simulink model "RefModel_2024"  (R2025b)
settings: Solver=VariableStepAuto  StartTime=0.0  StopTime=10.0  RelTol=1e-3
libraries: aerolibasang x3, simulink_extras x2, aerolibatmos2 x1
settings Model: Creator=Ranvir  LastModifiedBy=ranvirsingh

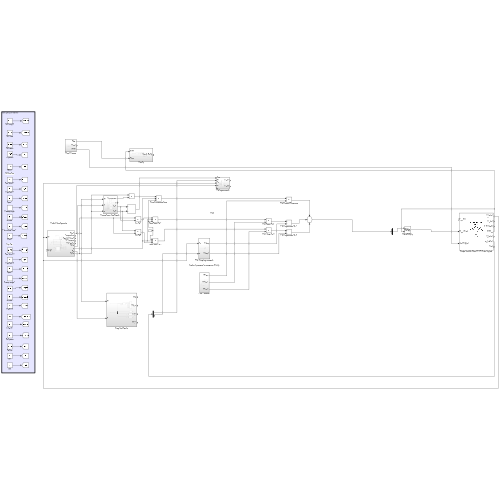
[thumbnail: Simulink's stored preview of the top-level diagram]
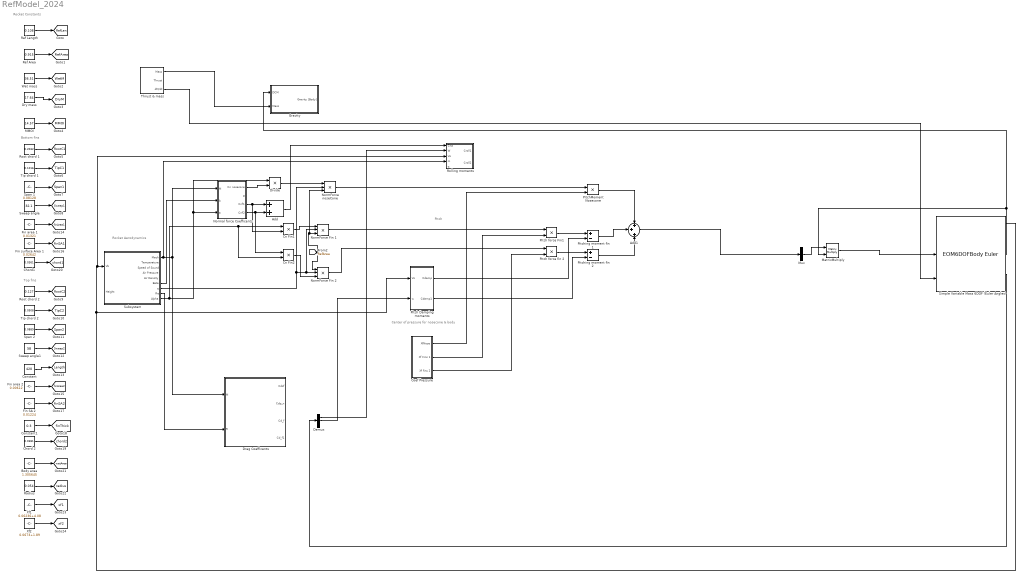
== system RefModel_2024 ==
  note: Center of pressure for nosecone & body
  note: Pitch
  note: Rocket Aerodynamics
  note: Bottom fins
  note: Rocket Constants
  note: Top fins
  Add : Sum
  Add1 : Sum  Inputs=+++
  Body area : Constant  Value=1.305645
  Chord 2 : Constant  Value=0.0381
  Chord1 : Constant  Value=0.0361
  Cn Fin1 : Product  Inputs=**
  Cn Fin2 : Product  Inputs=**
  Coef Pressure : Subsystem
  Constant : Constant  Value=420
  Constant1 : Constant  Value=0.3
  Demux : Demux  Outputs=3
  Divide : Product  Inputs=**
  Drag Coefficents : Subsystem
  Dry mass : Constant  Value=17.64
  Fin SA 2 : Constant  Value=0.01224
  Fin area 1 : Constant  Value=0.01321
  Fin area 2 : Constant  Value=0.00612
  Fin surface Area 1 : Constant  Value=0.02642
  Gravity : Subsystem
  MMOI : Constant  Value=14.57
  MatrixMultiply : Product  Multiplication=Matrix(*)
  Mux : Mux  Inputs=3
  NormForce Fin 1 : Product  Inputs=***
  NormForce Fin 2 : Product  Inputs=***
  NormForce noseCone : Product  Inputs=***
  Normal force Coefficents : Subsystem
  Pitch Damping moments : Subsystem
  Pitch force Fin1 : Product  Inputs=**
  Pitch force fin 2 : Product  Inputs=**
  PitchMoment Nosecone : Product  Inputs=**
  Pitching moment fin 1 : Sum  Inputs=+-
  Pitching moment fin 2 : Sum  Inputs=+-
  Radius : Constant  Value=0.054
  Ref Area : Constant  Value=0.915
  Ref Length : Constant  Value=0.108
  Rolling moments : Subsystem
  Root chord 1 : Constant  Value=0.2032
  Root chord 2 : Constant  Value=0.127
  Simple Variable Mass 6DOF (Euler Angles) : EOM6DOFBodyEuler  mtype=Simple Variable
  Span 1 : Constant  Value=0.08128
  Span 2 : Constant  Value=0.0889
  Subsystem : Subsystem
  Sweep angle : Constant  Value=32.1
  Sweep angle1 : Constant  Value=58
  Thrust & mass : Subsystem
  Tip chord 1 : Constant  Value=0.1016
  Tip chord 2 : Constant  Value=0.0508
  Wet mass : Constant  Value=36.51
  Xf1 : Constant  Value=0.06236+4.08
  Xf2 : Constant  Value=0.0673+1.89
  tag scope: DryM=global, Length=global, MMOI=global, RefArea=global, RefLen=global, RootC1=global, RootC2=global, Span1=global, Span2=global, Sweep1=global, Sweep2=global, TipC1=global, TipC2=global, WetM=global, chord1=global, chord2=global, finArea1=global, finArea2=global, finSA1=global, finSA2=global, finThick=global, radius=global, wetArea=global, xf1=global, xf2=global
  wires:
  Ref Length/1 -> [RefLen]
  Ref Area/1 -> [RefArea]
  Wet mass/1 -> [WetM]
  Dry mass/1 -> [DryM]
  MMOI/1 -> [MMOI]
  Root chord 1/1 -> [RootC1]
  Tip chord 1/1 -> [TipC1]
  Span 1/1 -> [Span1]
  Sweep angle/1 -> [Sweep1]
  Root chord 2/1 -> [RootC2]
  Tip chord 2/1 -> [TipC2]
  Span 2/1 -> [Span2]
  Sweep angle1/1 -> [Sweep2]
  Thrust & mass/1(Mass) -> Gravity/2(Mass)
  Simple Variable Mass 6DOF (Euler Angles)/4 -> MatrixMultiply/2, Gravity/1(DCM)
  Thrust & mass/3(dM/dt) -> Simple Variable Mass 6DOF (Euler Angles)/3
  Constant/1 -> [Length]
  Simple Variable Mass 6DOF (Euler Angles)/1 -> Pitch Damping moments/1(Vo), Rolling moments/3(Vo), Subsystem/1(Vb)
  Fin area 1/1 -> [finArea1]
  Fin area 2/1 -> [finArea2]
  Fin surface Area 1/1 -> [finSA1]
  Fin SA 2/1 -> [finSA2]
  Subsystem/1(Mach) -> Rolling moments/4(m), Drag Coefficents/1(M), Normal force Coefficents/1(M)
  Constant1/1 -> [finThick]
  Chord 2/1 -> [chord2]
  Chord1/1 -> [chord1]
  Body area/1 -> [wetArea]
  Subsystem/8(Re) -> Drag Coefficents/2(R)
  Subsystem/6(Beta) -> Normal force Coefficents/2(b)
  Subsystem/9(Alpha) -> Cn Fin2/2, Cn Fin1/1, Divide/1, Normal force Coefficents/3(a)
  Normal force Coefficents/3(Cnf1) -> Cn Fin1/2, Add/1
  Normal force Coefficents/4(Cnf2) -> Cn Fin2/1, Add/2
  Radius/1 -> [radius]
  Add/1 -> Rolling moments/1(Cna)
  Simple Variable Mass 6DOF (Euler Angles)/6 -> Demux/1
  Xf1/1 -> [xf1]
  Xf2/1 -> [xf2]
  Demux/1 -> Rolling moments/2(W)
  Cn Fin1/1 -> NormForce Fin 1/1
  [RefArea] -> NormForce noseCone/3, NormForce Fin 1/3, NormForce Fin 2/1
  Subsystem/7(q) -> NormForce Fin 1/2, NormForce Fin 2/2, NormForce noseCone/2
  Cn Fin2/1 -> NormForce Fin 2/3
  NormForce Fin 1/1 -> Pitch force Fin1/1
  NormForce Fin 2/1 -> Pitch force fin 2/1
  Normal force Coefficents/1(Cn nosecone) -> Divide/2
  Divide/1 -> NormForce noseCone/1
  NormForce noseCone/1 -> PitchMoment Nosecone/1
  Pitch force Fin1/1 -> Pitching moment fin 1/1
  Pitch force fin 2/1 -> Pitching moment fin 2/1
  Pitching moment fin 2/1 -> Add1/3
  Pitching moment fin 1/1 -> Add1/2
  PitchMoment Nosecone/1 -> Add1/1
  Add1/1 -> Mux/2
  Mux/1 -> MatrixMultiply/1
  MatrixMultiply/1 -> Simple Variable Mass 6DOF (Euler Angles)/2
  Coef Pressure/1(XfNose) -> PitchMoment Nosecone/2
  Coef Pressure/2(Xf Fins 1) -> Pitch force Fin1/2
  Coef Pressure/3(Xf fins 2) -> Pitch force fin 2/2
  Demux/2 -> Pitch Damping moments/2(w)
  Pitch Damping moments/1(Cdamp) -> Pitching moment fin 1/2
  Pitch Damping moments/2(Cdamp1) -> Pitching moment fin 2/2

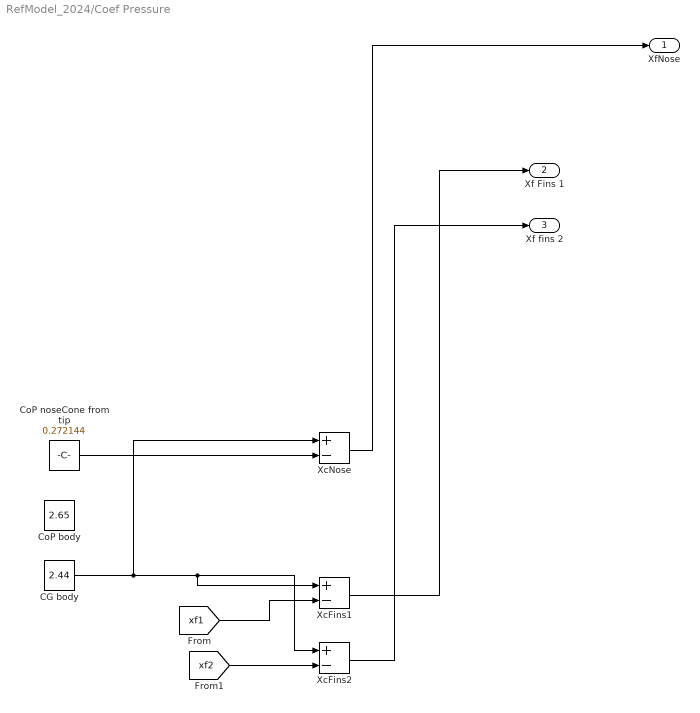
== system RefModel_2024/Coef Pressure ==
  CG body : Constant  Value=2.44
  CoP body : Constant  Value=2.65
  CoP noseCone from tip : Constant  Value=0.272144
  XcFins1 : Sum  Inputs=+-
  XcFins2 : Sum  Inputs=+-
  XcNose : Sum  Inputs=+-
  XfNose : Outport
  Xf Fins 1 : Outport  Port=2
  Xf fins 2 : Outport  Port=3
  wires:
  XcFins1/1 -> Xf Fins 1/1
  CoP noseCone from tip/1 -> XcNose/2
  CG body/1 -> XcNose/1, XcFins2/1, XcFins1/1
  [xf2] -> XcFins2/2
  [xf1] -> XcFins1/2
  XcFins2/1 -> Xf fins 2/1
  XcNose/1 -> XfNose/1

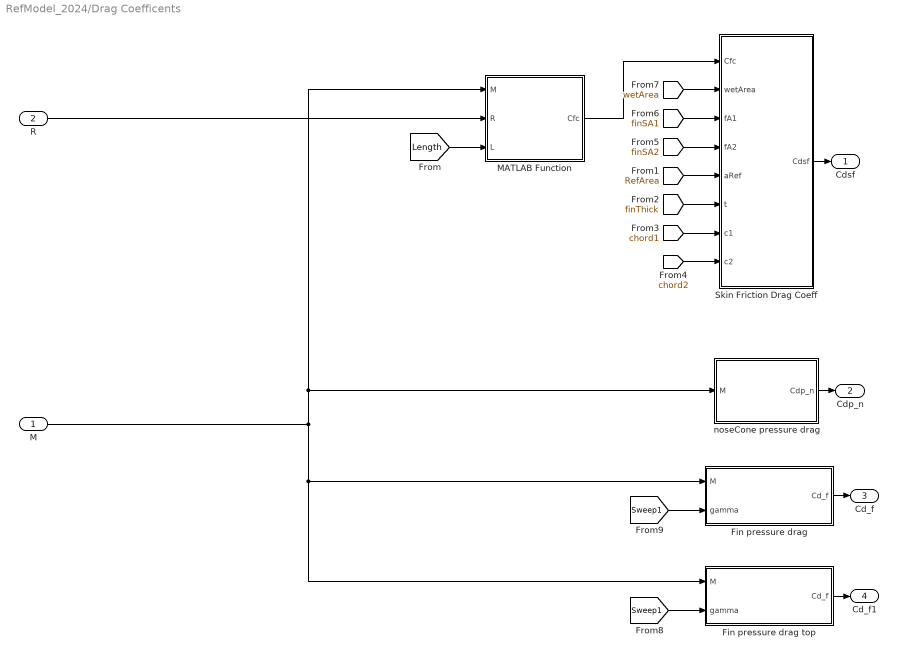
== system RefModel_2024/Drag Coefficents ==
  M : Inport
  R : Inport  Port=2
  Fin pressure drag : MATLAB Function  TreatAsAtomicUnit=on
  Fin pressure drag top : MATLAB Function  TreatAsAtomicUnit=on
  MATLAB Function : MATLAB Function  TreatAsAtomicUnit=on
  Skin Friction Drag Coeff : MATLAB Function  TreatAsAtomicUnit=on
  noseCone pressure drag : MATLAB Function  TreatAsAtomicUnit=on
  Cdsf : Outport
  Cdp_n : Outport  Port=2
  Cd_f : Outport  Port=3
  Cd_f1 : Outport  Port=4
  wires:
  MATLAB Function/1(Cfc) -> Skin Friction Drag Coeff/1(Cfc)
  [finSA2] -> Skin Friction Drag Coeff/4(fA2)
  M/1 -> MATLAB Function/1(M), noseCone pressure drag/1(M), Fin pressure drag top/1(M), Fin pressure drag/1(M)
  [finThick] -> Skin Friction Drag Coeff/6(t)
  Fin pressure drag/1(Cd_f) -> Cd_f/1
  [Sweep1] -> Fin pressure drag top/2(gamma)
  [Length] -> MATLAB Function/3(L)
  [Sweep1] -> Fin pressure drag/2(gamma)
  [finSA1] -> Skin Friction Drag Coeff/3(fA1)
  [chord2] -> Skin Friction Drag Coeff/8(c2)
  [wetArea] -> Skin Friction Drag Coeff/2(wetArea)
  [RefArea] -> Skin Friction Drag Coeff/5(aRef)
  [chord1] -> Skin Friction Drag Coeff/7(c1)
  R/1 -> MATLAB Function/2(R)
  noseCone pressure drag/1(Cdp_n) -> Cdp_n/1
  Fin pressure drag top/1(Cd_f) -> Cd_f1/1
  Skin Friction Drag Coeff/1(Cdsf) -> Cdsf/1

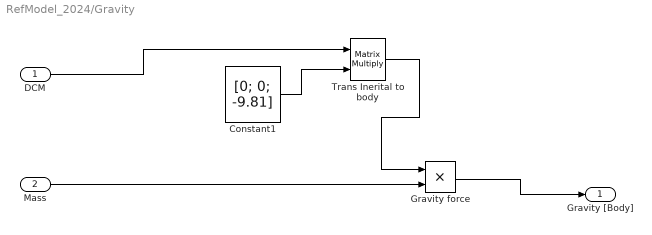
== system RefModel_2024/Gravity ==
  DCM : Inport
  Mass : Inport  Port=2
  Constant1 : Constant  Value=[0; 0; -9.81]  VectorParams1D=off
  Gravity force : Product  Inputs=**
  Trans Inerital to body : Product  Multiplication=Matrix(*)
  Gravity [Body] : Outport
  wires:
  Constant1/1 -> Trans Inerital to body/2
  Trans Inerital to body/1 -> Gravity force/1
  Mass/1 -> Gravity force/2
  Gravity force/1 -> Gravity [Body]/1
  DCM/1 -> Trans Inerital to body/1

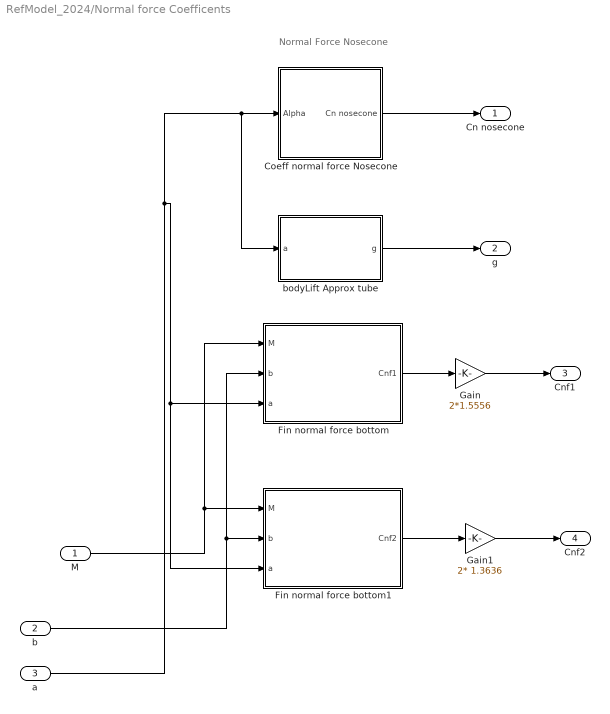
== system RefModel_2024/Normal force Coefficents ==
  note: Normal Force Nosecone
  M : Inport
  b : Inport  Port=2
  a : Inport  Port=3
  Coeff normal force Nosecone : Subsystem
  Fin normal force bottom : Subsystem
  Fin normal force bottom1 : Subsystem
  Gain : Gain  Gain=2*1.5556
  Gain1 : Gain  Gain=2* 1.3636
  bodyLift Approx tube : MATLAB Function  TreatAsAtomicUnit=on
  Cn nosecone : Outport
  g : Outport  Port=2
  Cnf1 : Outport  Port=3
  Cnf2 : Outport  Port=4
  wires:
  M/1 -> Fin normal force bottom/1(M), Fin normal force bottom1/1(M)
  a/1 -> Fin normal force bottom1/3(a), Fin normal force bottom/3(a), bodyLift Approx tube/1(a), Coeff normal force Nosecone/1(Alpha)
  Coeff normal force Nosecone/1(Cn nosecone) -> Cn nosecone/1
  bodyLift Approx tube/1(g) -> g/1
  b/1 -> Fin normal force bottom/2(b), Fin normal force bottom1/2(b)
  Fin normal force bottom1/1(Cnf2) -> Gain1/1
  Fin normal force bottom/1(Cnf1) -> Gain/1
  Gain/1 -> Cnf1/1
  Gain1/1 -> Cnf2/1

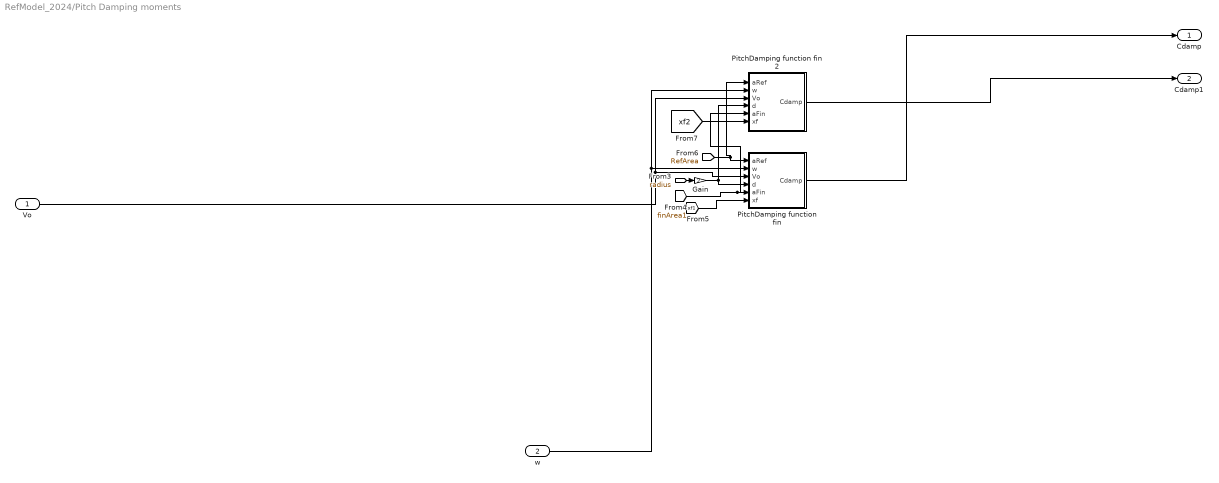
== system RefModel_2024/Pitch Damping moments ==
  Vo : Inport
  w : Inport  Port=2
  Gain : Gain  Gain=2
  PitchDamping function fin : MATLAB Function  TreatAsAtomicUnit=on
  PitchDamping function fin 2 : MATLAB Function  TreatAsAtomicUnit=on
  Cdamp : Outport
  Cdamp1 : Outport  Port=2
  wires:
  w/1 -> PitchDamping function fin 2/2(w), PitchDamping function fin/2(w)
  PitchDamping function fin 2/1(Cdamp) -> Cdamp1/1
  [xf1] -> PitchDamping function fin/6(xf)
  [finArea1] -> PitchDamping function fin 2/5(aFin), PitchDamping function fin/5(aFin)
  [radius] -> Gain/1
  Gain/1 -> PitchDamping function fin 2/4(d), PitchDamping function fin/4(d)
  [xf2] -> PitchDamping function fin 2/6(xf)
  [RefArea] -> PitchDamping function fin 2/1(aRef), PitchDamping function fin/1(aRef)
  Vo/1 -> PitchDamping function fin 2/3(Vo), PitchDamping function fin/3(Vo)
  PitchDamping function fin/1(Cdamp) -> Cdamp/1

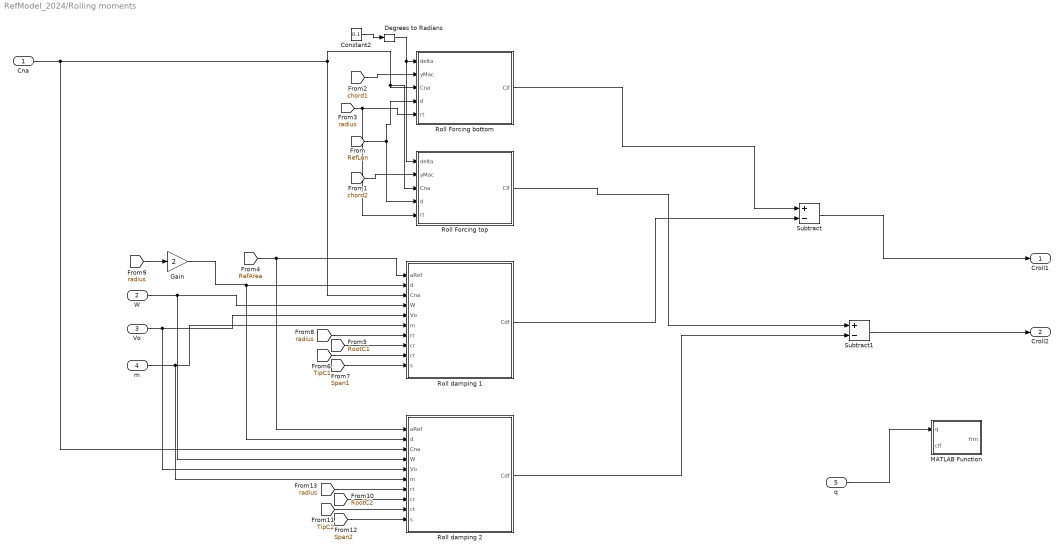
== system RefModel_2024/Rolling moments ==
  Cna : Inport
  W : Inport  Port=2
  Vo : Inport  Port=3
  m : Inport  Port=4
  q : Inport  Port=5
  Constant2 : Constant  Value=0.1
  Degrees to Radians : simulink_extras/Transformations/Degrees to Radians
  Gain : Gain  Gain=2
  MATLAB Function : MATLAB Function  TreatAsAtomicUnit=on
  Roll Forcing bottom : MATLAB Function  TreatAsAtomicUnit=on
  Roll Forcing top : MATLAB Function  TreatAsAtomicUnit=on
  Roll damping 1 : MATLAB Function  TreatAsAtomicUnit=on
  Roll damping 2 : MATLAB Function  TreatAsAtomicUnit=on
  Subtract : Sum  Inputs=+-
  Subtract1 : Sum  Inputs=+-
  Croll1 : Outport
  Croll2 : Outport  Port=2
  wires:
  Constant2/1 -> Degrees to Radians/1
  Cna/1 -> Roll damping 2/3(Cna), Roll Forcing top/3(Cna), Roll Forcing bottom/3(Cna), Roll damping 1/3(Cna)
  [RefLen] -> Roll Forcing bottom/4(d), Roll Forcing top/4(d)
  [radius] -> Roll Forcing top/5(rt), Roll Forcing bottom/5(rt)
  [chord1] -> Roll Forcing bottom/2(yMac)
  Degrees to Radians/1 -> Roll Forcing top/1(delta), Roll Forcing bottom/1(delta)
  [chord2] -> Roll Forcing top/2(yMac)
  Roll Forcing top/1(Clf) -> Subtract1/1
  Roll Forcing bottom/1(Clf) -> Subtract/1
  [RefArea] -> Roll damping 2/1(aRef), Roll damping 1/1(aRef)
  [radius] -> Roll damping 1/7(rt)
  [RootC1] -> Roll damping 1/8(cr)
  [TipC1] -> Roll damping 1/9(ct)
  [Span1] -> Roll damping 1/10(s)
  [radius] -> Gain/1
  W/1 -> Roll damping 2/4(W), Roll damping 1/4(W)
  Vo/1 -> Roll damping 2/5(Vo), Roll damping 1/5(Vo)
  m/1 -> Roll damping 2/6(m), Roll damping 1/6(m)
  [radius] -> Roll damping 2/7(rt)
  [Span2] -> Roll damping 2/10(s)
  [TipC2] -> Roll damping 2/9(ct)
  [RootC2] -> Roll damping 2/8(cr)
  Roll damping 1/1(Cdf) -> Subtract/2
  Roll damping 2/1(Cdf) -> Subtract1/2
  Subtract/1 -> Croll1/1
  Subtract1/1 -> Croll2/1
  Gain/1 -> Roll damping 2/2(d), Roll damping 1/2(d)
  q/1 -> MATLAB Function/1(q)

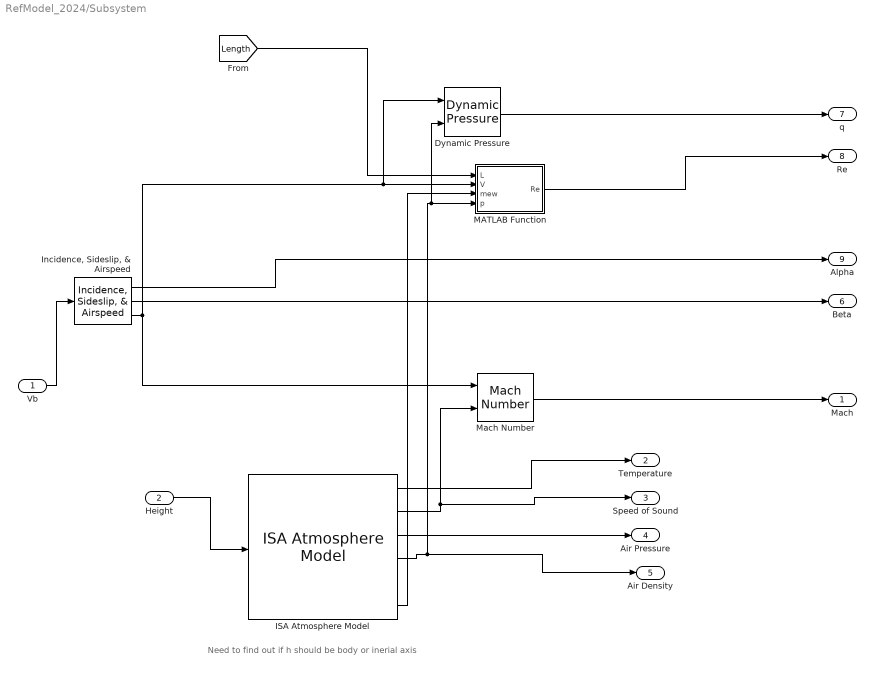
== system RefModel_2024/Subsystem ==
  note: Need to find out if h should be body or inerial axis
  Vb : Inport
  Height : Inport  Port=2
  Dynamic Pressure : aerolibasang/Dynamic Pressure
  ISA Atmosphere Model : aerolibatmos2/ISA Atmosphere Model  useExtended=off  action=None  custom=off  viscosityOut=on  g=9.80665  gamma=1.4  R=287.0531  L=0.0065  h_trop=11000  h_strat=20000  rho0=1.225  P0=101325  T0=288.15  h0=0  S=110.4  Tref=273.15  muref=1.716e-5
  "Incidence, Sideslip, & Airspeed" : aerolibasang/Incidence, Sideslip, & Airspeed
  MATLAB Function : MATLAB Function  TreatAsAtomicUnit=on
  Mach Number : aerolibasang/Mach Number
  Mach : Outport
  Temperature : Outport  Port=2
  Speed of Sound : Outport  Port=3
  Air Pressure : Outport  Port=4
  Air Density : Outport  Port=5
  Beta : Outport  Port=6
  q : Outport  Port=7
  Re : Outport  Port=8
  Alpha : Outport  Port=9
  wires:
  Mach Number/1 -> Mach/1
  Height/1 -> ISA Atmosphere Model/1
  ISA Atmosphere Model/2 -> Mach Number/2, Speed of Sound/1
  ISA Atmosphere Model/3 -> Air Pressure/1
  ISA Atmosphere Model/1 -> Temperature/1
  ISA Atmosphere Model/4 -> Dynamic Pressure/2, MATLAB Function/4(p), Air Density/1
  "Incidence, Sideslip, & Airspeed"/2 -> Beta/1
  "Incidence, Sideslip, & Airspeed"/1 -> Alpha/1
  Vb/1 -> "Incidence, Sideslip, & Airspeed"/1
  "Incidence, Sideslip, & Airspeed"/3 -> Dynamic Pressure/1, MATLAB Function/2(V), Mach Number/1
  [Length] -> MATLAB Function/1(L)
  MATLAB Function/1(Re) -> Re/1
  ISA Atmosphere Model/6 -> MATLAB Function/3(mew)
  Dynamic Pressure/1 -> q/1

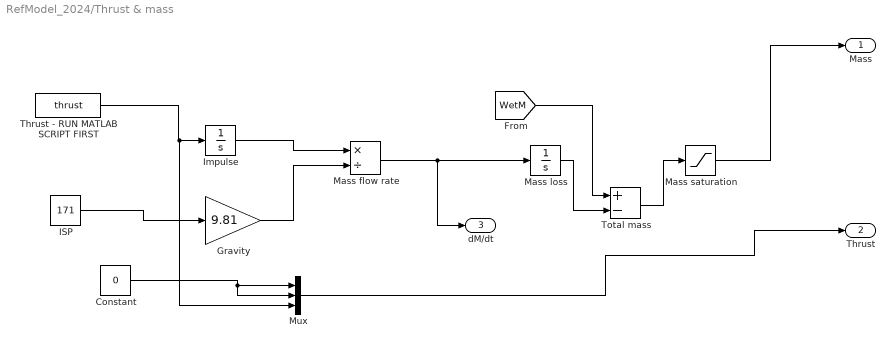
== system RefModel_2024/Thrust & mass ==
  Constant : Constant  Value=0
  Gravity : Gain  Gain=9.81
  ISP : Constant  Value=171
  Impulse : Integrator
  Mass flow rate : Product  Inputs=*/
  Mass loss : Integrator  UpperSaturationLimit=7  LowerSaturationLimit=0
  Mass saturation : Saturate  UpperLimit=36.51  LowerLimit=17.64
  Mux : Mux  Inputs=3
  Thrust - RUN MATLAB SCRIPT FIRST : FromWorkspace  VariableName=thrust  OutputAfterFinalValue=Setting to zero
  Total mass : Sum  Inputs=+-
  Mass : Outport
  Thrust : Outport  Port=2
  dM/dt : Outport  Port=3
  wires:
  Thrust - RUN MATLAB SCRIPT FIRST/1 -> Mux/3, Impulse/1
  Total mass/1 -> Mass saturation/1
  Gravity/1 -> Mass flow rate/2
  Mass flow rate/1 -> dM/dt/1, Mass loss/1
  [WetM] -> Total mass/1
  ISP/1 -> Gravity/1
  Impulse/1 -> Mass flow rate/1
  Mass loss/1 -> Total mass/2
  Mass saturation/1 -> Mass/1
  Constant/1 -> Mux/2, Mux/1
  Mux/1 -> Thrust/1

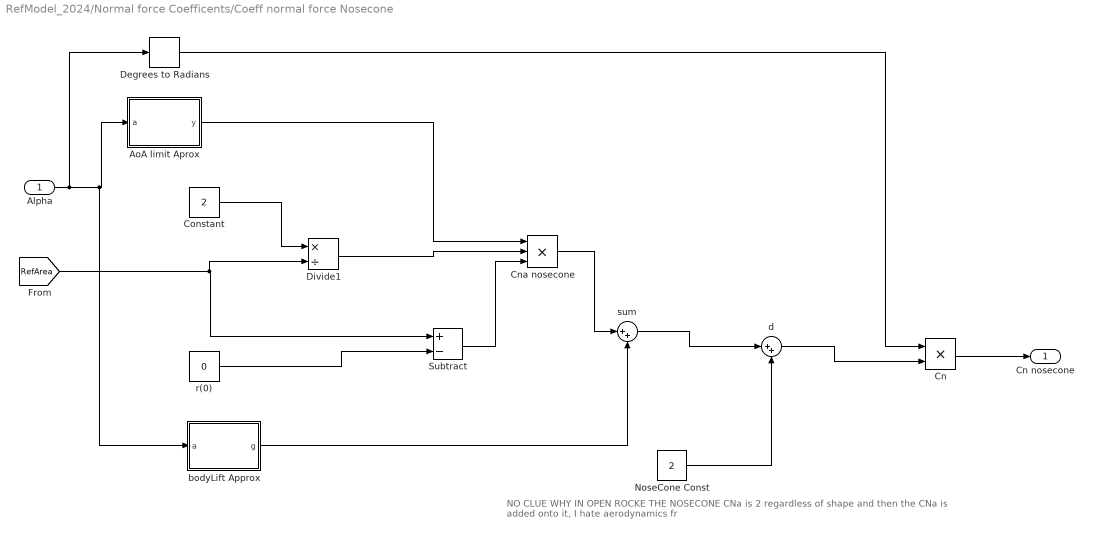
== system RefModel_2024/Normal force Coefficents/Coeff normal force Nosecone ==
  note: NO CLUE WHY IN OPEN ROCKE THE NOSECONE CNa is 2 regardless of shape and then the CNa is added onto it, I hate aerodynamics fr
  Alpha : Inport
  AoA limit Aprox : MATLAB Function  TreatAsAtomicUnit=on
  Cn : Product  Inputs=**
  Cna nosecone : Product  Inputs=***
  Constant : Constant  Value=2
  Degrees to Radians : simulink_extras/Transformations/Degrees to Radians
  Divide1 : Product  Inputs=*/
  NoseCone Const : Constant  Value=2
  Subtract : Sum  Inputs=+-
  bodyLift Approx : MATLAB Function  TreatAsAtomicUnit=on
  d : Sum  Inputs=|++
  r(0) : Constant  Value=0
  sum : Sum  Inputs=|++
  Cn nosecone : Outport
  wires:
  [RefArea] -> Divide1/2, Subtract/1
  Cna nosecone/1 -> sum/1
  sum/1 -> d/1
  Subtract/1 -> Cna nosecone/3
  bodyLift Approx/1(g) -> sum/2
  Constant/1 -> Divide1/1
  AoA limit Aprox/1(y) -> Cna nosecone/1
  Alpha/1 -> Degrees to Radians/1, bodyLift Approx/1(a), AoA limit Aprox/1(a)
  Divide1/1 -> Cna nosecone/2
  r(0)/1 -> Subtract/2
  NoseCone Const/1 -> d/2
  Degrees to Radians/1 -> Cn/1
  d/1 -> Cn/2
  Cn/1 -> Cn nosecone/1

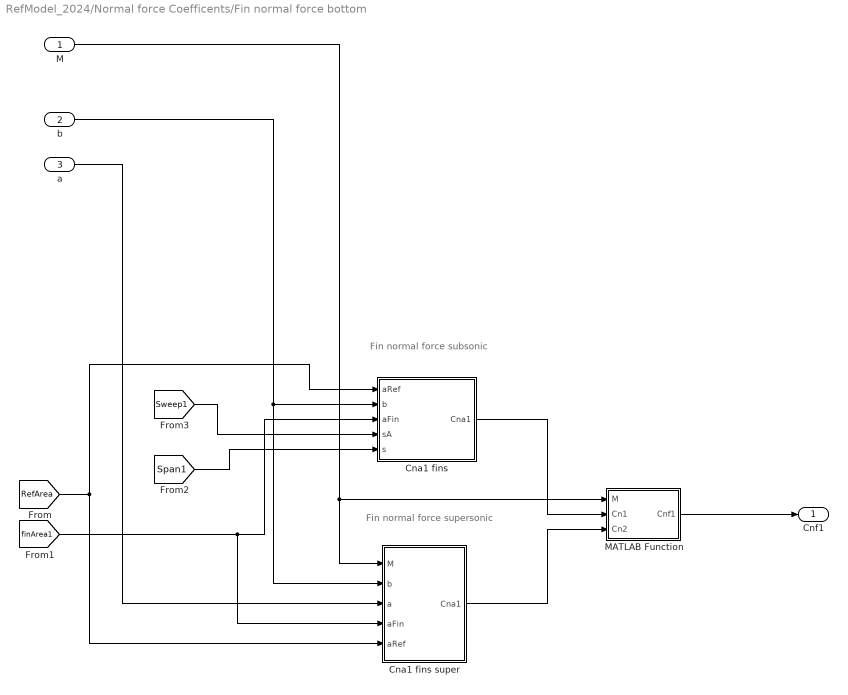
== system RefModel_2024/Normal force Coefficents/Fin normal force bottom ==
  note: Fin normal force supersonic
  note: Fin normal force subsonic
  M : Inport
  b : Inport  Port=2
  a : Inport  Port=3
  Cna1 fins : MATLAB Function  TreatAsAtomicUnit=on
  Cna1 fins super : MATLAB Function  TreatAsAtomicUnit=on
  MATLAB Function : MATLAB Function  TreatAsAtomicUnit=on
  Cnf1 : Outport
  wires:
  a/1 -> Cna1 fins super/3(a)
  [Sweep1] -> Cna1 fins/4(sA)
  [RefArea] -> Cna1 fins/1(aRef), Cna1 fins super/5(aRef)
  b/1 -> Cna1 fins super/2(b), Cna1 fins/2(b)
  [finArea1] -> Cna1 fins/3(aFin), Cna1 fins super/4(aFin)
  [Span1] -> Cna1 fins/5(s)
  M/1 -> MATLAB Function/1(M), Cna1 fins super/1(M)
  Cna1 fins super/1(Cna1) -> MATLAB Function/3(Cn2)
  Cna1 fins/1(Cna1) -> MATLAB Function/2(Cn1)
  MATLAB Function/1(Cnf1) -> Cnf1/1

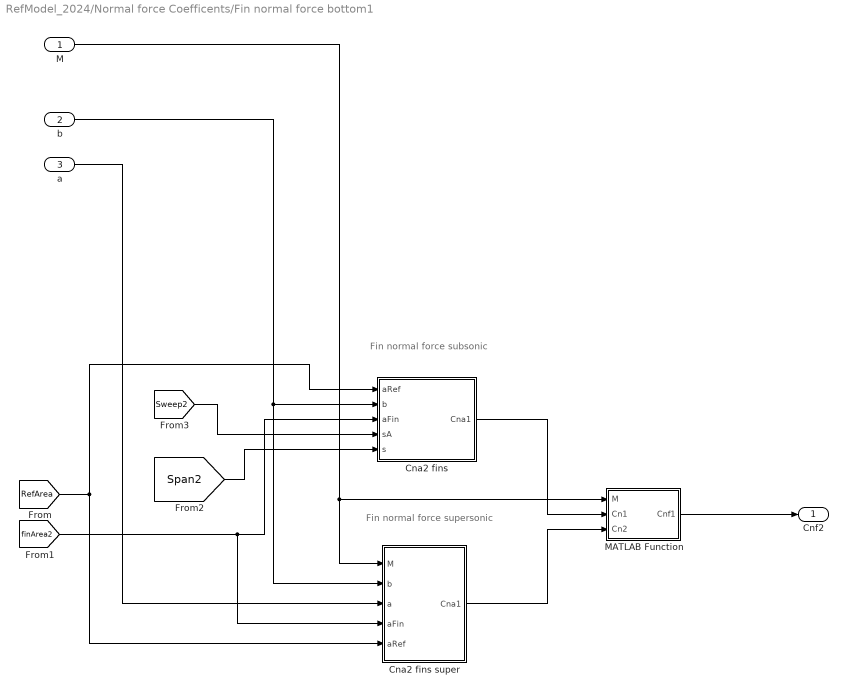
== system RefModel_2024/Normal force Coefficents/Fin normal force bottom1 ==
  note: Fin normal force supersonic
  note: Fin normal force subsonic
  M : Inport
  b : Inport  Port=2
  a : Inport  Port=3
  Cna2 fins : MATLAB Function  TreatAsAtomicUnit=on
  Cna2 fins super : MATLAB Function  TreatAsAtomicUnit=on
  MATLAB Function : MATLAB Function  TreatAsAtomicUnit=on
  Cnf2 : Outport
  wires:
  a/1 -> Cna2 fins super/3(a)
  [Sweep2] -> Cna2 fins/4(sA)
  [RefArea] -> Cna2 fins/1(aRef), Cna2 fins super/5(aRef)
  b/1 -> Cna2 fins super/2(b), Cna2 fins/2(b)
  [finArea2] -> Cna2 fins/3(aFin), Cna2 fins super/4(aFin)
  [Span2] -> Cna2 fins/5(s)
  M/1 -> MATLAB Function/1(M), Cna2 fins super/1(M)
  Cna2 fins super/1(Cna1) -> MATLAB Function/3(Cn2)
  Cna2 fins/1(Cna1) -> MATLAB Function/2(Cn1)
  MATLAB Function/1(Cnf1) -> Cnf2/1

== matlab function RefModel_2024/Normal force Coefficents/Fin normal force bottom1/MATLAB Function ==
  data: M input; Cnf1 output; Cn1 input; Cn2 input
function Cnf1 = fcn(M, Cn1, Cn2)

if M >=1
    Cnf1 = Cn2;
else
    Cnf1 = Cn1;
end

== matlab function RefModel_2024/Drag Coefficents/MATLAB Function ==
  data: M input; Cfc output; R input; L input
function Cfc = fcn(M,R, L)

Rs = 20;

Rcrit = 51*(Rs/L)^-1.039;


if R < 1*10^4
    Cfc = 1.48*10^-2;
elseif R < Rcrit
    cf = 1/((1.5*log(R) -5.6)^2);
    
    if M >= 1
        Cfc = cf/((1+0.15*M^2)^0.58);
    else
        Cfc = cf*(1-0.1*M^2);
    end

else
    cf = 0.032*(Rs/L)^0.2;

    if M >= 1
        Cfc = cf/(1+0.18*M^2);
    else
        Cfc = cf*(1-0.1*M^2);
    end

end

== matlab function RefModel_2024/Drag Coefficents/Skin Friction Drag Coeff ==
  data: Cfc input; Cdsf output; wetArea input; fA1 input; fA2 input; aRef input; t input; c1 input; c2 input
function Cdsf = fcn(Cfc, wetArea, fA1, fA2, aRef, t, c1, c2)

fb = 38.89;




top1 = (1+1/(2*fb)*wetArea);
top2 = (1+((2*t)/(c1)))*fA1;
top3 = (1+((2*t)/(c2)))*fA2;

Cdsf = Cfc*((top1+top2 + top3))/aRef;

== matlab function RefModel_2024/Drag Coefficents/noseCone pressure drag ==
  data: M input; Cdp_n output
function Cdp_n = fcn(M)



Fn = 2.42;
epsilon = atan(1/(2*Fn));

if M > 1.3
    Cdp_n = 2.1*(sin(epsilon))^2 + 0.5*((sin(epsilon))/(sqrt(M^2-1)));
elseif M > 1
    Cdp_n =0.8*sin(deg2rad(30))^2;
elseif M == 1
    Cdp_n = sin(epsilon);
else 

    y1 =0.8*sin(deg2rad(30))^2;
    y2 = sin(epsilon);

    Cdp_n = (y1*(1.3 - M) + y2*(M-0))/(1.3);
    

end

== matlab function RefModel_2024/Drag Coefficents/Fin pressure drag ==
  data: M input; Cd_f output; gamma input
function Cd_f = fcn(M, gamma)


Cd_TE = 0; % assuming taper trailing edge

if M < 0.9
    Cd_LE = (1-M^2)^(-0.417) - 1;
elseif M>=0.9 && M<1
   Cd_LE = 1-1.785*(M-0.9);
else
    Cd_LE = 1.214-((0.502)/(M^2))+((0.1095)/(M^4));
end

Cd_LEgam = Cd_LE*(cosd(gamma))^2;

Cd_f = Cd_LEgam + Cd_TE;

== matlab function RefModel_2024/Drag Coefficents/Fin pressure drag top ==
  data: M input; Cd_f output; gamma input
function Cd_f = fcn(M, gamma)


Cd_TE = 0; % assuming taper trailing edge

if M < 0.9
    Cd_LE = (1-M^2)^(-0.417) - 1;
elseif M>=0.9 && M<1
   Cd_LE = 1-1.785*(M-0.9);
else
    Cd_LE = 1.214-((0.502)/(M^2))+((0.1095)/(M^4));
end

Cd_LEgam = Cd_LE*(cosd(gamma))^2;

Cd_f = Cd_LEgam + Cd_TE;

== matlab function RefModel_2024/Rolling moments/Roll Forcing bottom ==
  data: delta input; yMac input; Clf output; Cna input; d input; rt input
function Clf = fcn(delta, yMac, Cna, d, rt)


N = 4;

Clf = (N*(yMac + rt)*Cna*delta)/d;

== matlab function RefModel_2024/Normal force Coefficents/Coeff normal force Nosecone/bodyLift Approx ==
  data: a input; g output
function g = fcn(a)

g = 1.1*(0.263603/0.019)*sind(a)^2;

== matlab function RefModel_2024/Rolling moments/Roll Forcing top ==
  data: delta input; yMac input; Clf output; Cna input; d input; rt input
function Clf = fcn(delta, yMac, Cna, d, rt)


N = 3;

Clf = (N*(yMac + rt)*Cna*delta)/d;

== matlab function RefModel_2024/Rolling moments/Roll damping 1 ==
  data: aRef input; d input; Cna input; W input; Cdf output; Vo input; m input; rt input; cr input; ct input; s input
function Cdf = fcn(aRef, d, Cna, W, Vo, m, rt,cr,ct,s)


v = norm(Vo);

strip = (((cr+ct)/2)*rt^2*s) + (((cr+(2*ct))/3)*rt*s^2) + (((cr+(3*ct))/12)*s^3);

Cdf = 0.01;

if m >= 1
    Cdf = strip*((4)/(aRef*d));
elseif m < 1
    Cdf = strip*((4*Cna*W)/(aRef*d*v));
else
    Cdf =0.01;
end

== matlab function RefModel_2024/Pitch Damping moments/PitchDamping function fin 2 ==
  data: aRef input; Cdamp output; w input; Vo input; d input; aFin input; xf input
function Cdamp = fcn(aRef, w,Vo, d, aFin,xf)

v = norm(Vo);


zeta = xf - 2.44;

Cdamp = 0.6*((4*aFin*zeta^3)/(aRef*d)) * (w^2/v^2);

== matlab function RefModel_2024/Pitch Damping moments/PitchDamping function fin ==
  data: aRef input; Cdamp output; w input; Vo input; d input; aFin input; xf input
function Cdamp = fcn(aRef, w,Vo, d, aFin,xf)

v = norm(Vo);


zeta = xf - 2.44;

Cdamp = 0.6*((4*aFin*zeta^3)/(aRef*d)) * (w^2/v^2);

== matlab function RefModel_2024/Rolling moments/MATLAB Function ==
  data: q input; frm output; clf input
function frm = fcn(q, clf)

frm = u;

== matlab function RefModel_2024/Rolling moments/Roll damping 2 ==
  data: aRef input; d input; Cna input; W input; Cdf output; Vo input; m input; rt input; cr input; ct input; s input
function Cdf = fcn(aRef, d, Cna, W, Vo, m, rt,cr,ct,s)


v = norm(Vo);

strip = (((cr+ct)/2)*rt^2*s) + (((cr+(2*ct))/3)*rt*s^2) + (((cr+(3*ct))/12)*s^3);

Cdf = 0.01;

if m >= 1
    Cdf = strip*((4)/(aRef*d));
elseif m < 1
    Cdf = strip*((4*Cna*W)/(aRef*d*v));
else
    Cdf =0.01;
end

== matlab function RefModel_2024/Normal force Coefficents/Coeff normal force Nosecone/AoA limit Aprox ==
  data: a input; y output
function y = fcn(a)

if a == 0
    y = 1;
else
    y = sind(a)/a;
end

== matlab function RefModel_2024/Subsystem/MATLAB Function ==
  data: L input; Re output; V input; mew input; p input
function Re = fcn(L, V, mew, p)

Re = (L*V*p)/mew;

== matlab function RefModel_2024/Normal force Coefficents/bodyLift Approx tube ==
  data: a input; g output
function g = fcn(a)

g = 1.1*(0.263603/0.019)*sind(a)^2;

== matlab function RefModel_2024/Normal force Coefficents/Fin normal force bottom/Cna1 fins ==
  data: aRef input; Cna1 output; b input; aFin input; sA input; s input
function Cna1 = fcn(aRef, b, aFin,sA,s)



top = (2*pi) * ((s^2)/aRef);
fd = (b*s^2)/(aFin*cosd(sA)); 
bot = 1+sqrt(1+fd^2);


Cna1 = top/bot;

== matlab function RefModel_2024/Normal force Coefficents/Fin normal force bottom/Cna1 fins super ==
  data: M input; b input; a input; aFin input; aRef input; Cna1 output
% function Cna1 = fcn(M, b, a, aFin, aRef)
% 
% gam = 1.4;
% gam1 = gam+1;
% 
% k1 = 2/b;
% k2 = (gam1*(M^4) -(4*b^2))/(4*b^4);
% k3 = ( (gam1*M^8)  + ((2*gam^2 - 7*gam - 5)*M^6) + 10*(gam1)*M^4 + 8)/(6*b^7);
% 
% 
% 
% 
% 
% 
% Cna1 = (aFin/aRef) *(k1 + k2*a + k3*a^2);


function Cna1 = fcn(M, b, a, aFin, aRef)

s = 0.152; %m^2
 %m^2
sA = 30.8; %deg


top = (2*pi) * ((s^2)/aRef);
fd = (b*s^2)/(aFin*cosd(sA)); 
bot = 1+sqrt(1+fd^2);


Cna1 = top/bot;

== matlab function RefModel_2024/Normal force Coefficents/Fin normal force bottom/MATLAB Function ==
  data: M input; Cnf1 output; Cn1 input; Cn2 input
function Cnf1 = fcn(M, Cn1, Cn2)

if M >=1
    Cnf1 = Cn2;
else
    Cnf1 = Cn1;
end

== matlab function RefModel_2024/Normal force Coefficents/Fin normal force bottom1/Cna2 fins ==
  data: aRef input; Cna1 output; b input; aFin input; sA input; s input
function Cna1 = fcn(aRef, b, aFin,sA,s)



top = (2*pi) * ((s^2)/aRef);
fd = (b*s^2)/(aFin*cosd(sA)); 
bot = 1+sqrt(1+fd^2);


Cna1 = top/bot;

== matlab function RefModel_2024/Normal force Coefficents/Fin normal force bottom1/Cna2 fins super ==
  data: M input; b input; a input; aFin input; aRef input; Cna1 output
% function Cna1 = fcn(M, b, a, aFin, aRef)
% 
% gam = 1.4;
% gam1 = gam+1;
% 
% k1 = 2/b;
% k2 = (gam1*(M^4) -(4*b^2))/(4*b^4);
% k3 = ( (gam1*M^8)  + ((2*gam^2 - 7*gam - 5)*M^6) + 10*(gam1)*M^4 + 8)/(6*b^7);
% 
% 
% 
% 
% 
% 
% Cna1 = (aFin/aRef) *(k1 + k2*a + k3*a^2);


function Cna1 = fcn(M, b, a, aFin, aRef)

s = 0.152; %m^2
 %m^2
sA = 30.8; %deg


top = (2*pi) * ((s^2)/aRef);
fd = (b*s^2)/(aFin*cosd(sA)); 
bot = 1+sqrt(1+fd^2);


Cna1 = top/bot;
